simulink model "main_robot"  (R2025b)
settings: Solver=ode23t  StartTime=0.0  StopTime=120  RelTol=1e-3
InitFcn:
  | RPInit
model workspace (MAT data in the model file):
  mapForSim : object (value not decoded)
  occGrid : robotics.BinaryOccupancyGrid (value not decoded)
undefined symbols (not defined in the file or in its folder): Base, FloorSurface, PlowSurface, Ref, RobotSurface, Side1, Side2, X, Y, Z
libraries: sm_lib x27, nesl_utility x11, RP_Simulator_Components x7, ME598_ProjectLibrary x3, RoboticsPlayground x2
(part 2 of 2)

== matlab function main_robot/MATLAB Function ==
  data: redAngle input; redDistance input; leftMotor output; rightMotor output; greenAngle input; greenDistance input; blueAngle input; blueDistance input; debugVal output; robotX input; robotY input; robotAngle input; wallLeftDistance input; wallRightDistance input
function [leftMotor, rightMotor, debugVal] = main_robot( ...
    redAngle, ...
    redDistance, ...
    greenAngle, ...
    greenDistance, ...
    blueAngle, ...
    blueDistance, ...
    robotX, ...
    robotY, ...
    robotAngle, ...
    wallLeftDistance, ...
    wallRightDistance ...
    )

    % Robot States
    % 0 = Find closets roapmap point
    % 1 = Navigate to a point
    % 2 = Navigate over multiple points of a roadmap
    % 3 = something else

    % Object Colors
    % 0 = Red
    % 1 = Green
    % 2 = Blue

    function [leftMotor, rightMotor] = commandMotor(motion, distance)
        if motion == "spin-left"
            leftMotor = -30;
            rightMotor = 30;
        elseif motion == "spin-right"
            leftMotor = 30;
            rightMotor = -30;
        elseif motion == "stop"
            leftMotor = 0;
            rightMotor = 0;
        elseif motion == "forward"
            leftMotor = 75;
            rightMotor = 75;
        elseif motion == "forward-fast"
            leftMotor = 127;
            rightMotor = 127;
        elseif motion == "reverse"
            leftMotor = -75;
            rightMotor = -75;
        elseif motion == "swerve-right"
            leftMotor = 127;
            rightMotor = 127*distance/0.8;
        elseif motion == "swerve-left"
            leftMotor = 127*distance/0.8;
            rightMotor = 127;       
        end
    end

    persistent robotState
    %persistent objectLocationX
    %persistent objectLocationY
    persistent objectColor
    persistent currentObject
    persistent targetPositionsMatrix
    persistent targetPositionPointer
    persistent jobVector
    persistent jobVectorPointer
    persistent delivery
    persistent dropFlag
    persistent longDistanceTrip

    if isempty(robotState)
        %robotState = 1.11;
        robotState = 0;
    end
    %if isempty(objectLocationX)
    %    objectLocationX = -1.5;
    %end
    %if isempty(objectLocationY)
    %    objectLocationY = 0;
    %end
    if isempty(objectColor)
        objectColor = -1;
    end
    if isempty(currentObject)
        currentObject = 0;
    end
    if isempty(targetPositionsMatrix)
        %targetPositionsMatrix = zeros(1,2);
        %targetPositionsMatrix = zeros(2,2);
        targetPositionsMatrix = zeros(3,2);
    end    
    if isempty(targetPositionPointer)
        targetPositionPointer = 1;
    end
    if isempty(jobVector)
        jobVector = zeros(1,10);
    end    
    if isempty(jobVectorPointer)
        jobVectorPointer = 1;
    end
    if isempty(delivery)
        delivery = 0;
    end
    if isempty(dropFlag)
        dropFlag = 0;
    end
    if isempty(longDistanceTrip)
        longDistanceTrip = -1;
    end

    % Default values for all paths
    leftMotor  = 0;
    rightMotor = 0;
    debugVal = robotState;
    objectDistance = NaN;
    objectAngle = NaN;

    % Roadmap around object 0 (bottom)
    roadMapObject0 = [-0.3 -1.9; -1 -1.25; 0.75 -2.2];

    % Roadmap around object 1 (top)
    %roadMapObject1 = [-0.75 1.35; -0.6 1.97; 0.52 2.01]; 
    %roadMapObject1 = [-0.75 1.35; -0.5 1.97; 0.52 2.01]; %works for
    %blue-green
    
    % initial
    %roadMapObject1 = [-0.75 1.35; -0.5 2.1; 0.62 2.1]; 
    roadMapObject1 = [-0.75 1.35; -0.5 2.1; 0.52 2.01]; 

    % robotState 0: MAIN CONTROL
    % List of jobs:
    % 1 -> Determine closets point in roadmap
    % 2 -> Navigate to closest point
    % 3 -> Plan a Path from current position to collection zone
    % 4 -> Navigate to from current position to collection zone
    % 5 -> Determine disengage position
    % 6 -> Navigate to disengage position
    % 7 -
    
    if robotState == 0
        % is current job complete, move to next job
        if jobVector(1,jobVectorPointer)  
            jobVectorPointer = jobVectorPointer + 1
        end

        if jobVectorPointer == 1
            % determine closets point in roadmap
            robotState = 2

        elseif jobVectorPointer == 2
            % navigate to closest point
            robotState = 1.11
        elseif jobVectorPointer == 3
            % determine path 
            robotState = 3
        elseif jobVectorPointer == 4
            % Navigate to collection zone via roadmap
            delivery = 1
            robotState = 1.11
        elseif jobVectorPointer == 5
            %Determine disengage position
            robotState = 5
        elseif jobVectorPointer == 6
            % Navigate to disengage position
            robotState = 6
        elseif jobVectorPointer == 7
            pr = 'in job 7 main control--->'
            % Set a new system loop to operate on Object 1
            if currentObject == 0
                currentObject = 1
                jobVector = zeros(1,10);                    
                jobVectorPointer = 1
                robotState = 0
                longDistanceTrip = 1
            elseif currentObject == 1
                jobVector(1,jobVectorPointer) = 1;
            else
                error('currentObject must be 0 or 1')
            end
        elseif jobVectorPointer == 8
            % Set up home navigation
            robotState = 8
        elseif jobVectorPointer == 9
            % Navigate to home position
            longDistanceTrip = 1
            robotState = 1.11
        elseif jobVectorPointer == 10
            % Goal achieved. Do nothing.
            robotState = 9
        end

       
    end

    % robotState 1: Navigate to 1 or more points
    if robotState >= 1 && robotState < 2
        %targetPositionPointer
        xTarget = targetPositionsMatrix(targetPositionPointer,1)
        yTarget = targetPositionsMatrix(targetPositionPointer,2)
        longDistanceTrip
        % if longDistanceTrip has not been computed
        if longDistanceTrip == -1
            tripDistance = sqrt((robotX-xTarget)^2 + (robotY-yTarget)^2)
            if tripDistance >= 3.21
                longDistanceTrip = 1;
            else
                longDistanceTrip = 0;
            end
        end


        % robotState 1.1: Navigate to a point
        if robotState >= 1.1 && robotState < 1.2
            if robotState == 1.11
                % spin to find segment end         
                angleTarget = atan2d(yTarget - robotY, xTarget - robotX)
        
                if robotAngle > angleTarget - 2 && robotAngle < angleTarget + 2
                    [leftMotor, rightMotor] = commandMotor("stop");
                    robotState = 1.12
                else
                    % convert angles to a 0-360 range
                    ra = mod(robotAngle, 360);
                    ta = mod(angleTarget, 360);

                    angle_difference = mod((ta - ra + 180), 360) - 180;
                    
                    % Choose spin direction
                    if angle_difference > 0
                        [leftMotor, rightMotor] = commandMotor("spin-left");
                    elseif angle_difference < 0
                        [leftMotor, rightMotor] = commandMotor("spin-right");
                    else
                        % Already facing the target angle
                        [leftMotor, rightMotor] = commandMotor("stop");
                    end
                end
            end
        
            if robotState == 1.12
                % move to segment end
                if dropFlag == 1 || longDistanceTrip == 1
                    tolerance = 0.8;
                else
                    tolerance = 0.1;
                end
                if robotX > xTarget - tolerance && robotX < xTarget + tolerance && robotY > yTarget - tolerance && robotY < yTarget + tolerance
                    [leftMotor, rightMotor] = commandMotor("stop");
                    robotState = 1.2;
                else
                    if dropFlag == 1 && longDistanceTrip == 1
                        if wallLeftDistance <= 0.8
                            [leftMotor, rightMotor] = commandMotor("swerve-right", wallLeftDistance);
                        elseif wallRightDistance <= 0.8
                            [leftMotor, rightMotor] = commandMotor("swerve-left", wallRightDistance);
                        else
                            [leftMotor, rightMotor] = commandMotor("forward-fast");
                        end
                    elseif dropFlag == 1
                        [leftMotor, rightMotor] = commandMotor("forward-fast");
                    else
                        [leftMotor, rightMotor] = commandMotor("forward");
                    end
                end
            end

        end

        % robotState 1.2: increase pointer or finish navigation
        if robotState == 1.2
            % check there are pending location to visit 
            if size(targetPositionsMatrix,1) > targetPositionPointer
                targetPositionPointer = targetPositionPointer + 1
                longDistanceTrip = -1;
                % if this is the last segment of a delivery operation
                if targetPositionPointer == size(targetPositionsMatrix,1) && delivery == 1
                    dropFlag = 1;
                end
                robotState = 1.11
            else    % all positions have ben visited
                longDistanceTrip = -1;
                delivery = 0;
                dropFlag = 0;
                % reset targetPositionPointer
                targetPositionPointer = 1;
                % Mark current job as completed
                jobVector(1,jobVectorPointer) = 1;
                robotState = 0;
            end
        end
    end

    % robotstate 2: Find closest point in roadmap
    if robotState == 2
        pr = 'determining closest point'
        if currentObject == 0
            [x, y] = DETERMINE_CLOSEST_POINT(roadMapObject0, robotX, robotY);
        else
            [x, y] = DETERMINE_CLOSEST_POINT(roadMapObject1, robotX, robotY);
        end

        % set pointer to 2 so only the last x y is used
        targetPositionPointer = 3;
        targetPositionsMatrix = [0 0;0 0;x y];

        % Test moves for debugging
        %targetPositionsMatrix = [0 0; 0 0];
        %targetPositionsMatrix = [0 0; 2 -2];
        %targetPositionsMatrix = [-0.4 -2; 2 2.2];        % Arena(red, _)

        % Mark current job as completed
        jobVector(1, jobVectorPointer) = 1;
        robotState = 0;
    end

    % Robot looks for object. Spin until object found
    % Robots determines color of object. R: 1, G:2, B:3
    % Robot determines pre-plow position for the given color
    % Robot determines path to reach ppp and collection zone
    if robotState == 3
        if isnan(redDistance) && isnan(greenDistance) && isnan(blueDistance)
            if robotX < 0 && robotY < 0 || robotX < 0 && robotY > 0 
                % second or third quadrant
                [leftMotor, rightMotor] = commandMotor("spin-right");
            elseif robotX > 0 && robotY > 0
                % first quadrant
                [leftMotor, rightMotor] = commandMotor("spin-left");
            else
                [leftMotor, rightMotor] = commandMotor("spin-right");
            end
            
        else    % object detected
            [leftMotor, rightMotor] = commandMotor("stop");
            if ~isnan(redDistance)
                objectColor = 1
            elseif ~isnan(greenDistance)
                objectColor = 2
            elseif ~isnan(blueDistance)
                objectColor = 3
            else
                debugVal = -1;
            end

            % Determine pre-plow position for given color
            if currentObject == 0
                pppX = roadMapObject0(objectColor,1)
                pppY = roadMapObject0(objectColor,2)
                %[x, y] = DETERMINE_CLOSEST_POINT(roadMapObject0, robotX, robotY);
            else
                pppX = roadMapObject1(objectColor,1)
                pppY = roadMapObject1(objectColor,2)
                %[x, y] = DETERMINE_CLOSEST_POINT(roadMapObject1, robotX, robotY);
            end

            [targetPositionsMatrix, targetPositionPointer] = PATH_PLANNER(roadMapObject0, roadMapObject1, currentObject, objectColor, robotX, robotY, pppX, pppY)
            targetPositionsMatrix
            targetPositionPointer

            % Mark current job as completed
            pr = "Path planning"
            jobVector(1,jobVectorPointer) = 1;
            robotState = 0;

            return

        end
    end

    if robotState == 5 % WIP
        % calculate position that will create separation with object
        desired_separation = 0.5;
        x = robotX - desired_separation * cosd(robotAngle);
        y = robotY - desired_separation * sind(robotAngle);
    
        targetPositionsMatrix(3,1) = x;
        targetPositionsMatrix(3,2) = y;

        targetPositionPointer = 3;

        % Mark current job as completed
        jobVector(1,jobVectorPointer) = 1;
        robotState = 0;
    end
    
    % Navigate in reverse to disengage object
    if robotState == 6
        xTarget = targetPositionsMatrix(targetPositionPointer,1)
        yTarget = targetPositionsMatrix(targetPositionPointer,2)

        tolerance = 0.2;
        if robotX > xTarget - tolerance && robotX < xTarget + tolerance && robotY > yTarget - tolerance && robotY < yTarget + tolerance
            [leftMotor, rightMotor] = commandMotor("stop");
            pr = 'job 6 DONE'
            jobVector(1,jobVectorPointer) = 1;
            robotState = 0;            
        else
            [leftMotor, rightMotor] = commandMotor("reverse")
        end
    end

    if robotState == 8
   
        targetPositionsMatrix = [0 0;0 0;0 0]
        targetPositionPointer = 2;

        % Mark current job as completed
        jobVector(1,jobVectorPointer) = 1;
        robotState = 0;        
    end


end

== matlab function main_robot/-180* : 180* ==
  data: deg input; deg output
function deg = degWrap(deg)

% % Convert radians to degrees
% deg = 180/pi * rad;


% Wrap degree value to the range -180* : +180*
for idx = 1:length(deg)
    while deg(idx) < -180
        deg(idx) = deg(idx)+360;
    end
    
    while deg(idx) > 180
        deg(idx) = deg(idx)-360;
    end
end

return
